simulink model "buck_boost_SMC"  (R2025a)
settings: Solver=ode3  StartTime=0.0  StopTime=1  FixedStep=1e-3  RelTol=1e-3  EnableMultiTasking=on
values from neighbouring files (symbols this model uses):
  beta = 2e3    (= 2000)    [projeakt_3.m]
  C = 470*10^-6    (= 0.00047)    [projeakt_3.m]
  den_NF = [1/800 1]    [projeakt_3.m]
  E = 12    [projeakt_3.m]
  k0 = 4*30    (= 120)    [projeakt_3.m]
  k1 = 1    [projeakt_3.m]
  ki = 4*30^2    (= 3600)    [projeakt_3.m]
  L = Ls(i)*15.91e-3    [projeakt_3.m]
  noise_var = 0    [projeakt_3.m]
  num_NF = [1]    [projeakt_3.m]
  R = 52    [projeakt_3.m]
  sel = 3    [projeakt_3.m]
  x2e = Vc    (= -22.5)    [projeakt_3.m]
settings Model: Creator=Stevica  LastModifiedBy=PC
settings SolverCC: AlgebraicLoopSolver=TrustRegion
settings DataIOCC: LimitDataPoints=on  SaveFormat=Array  ReturnWorkspaceOutputs=off
settings OptimizationCC: LifeSpan=inf
settings DebuggingCC: UnderspecifiedInitializationDetection=Classic  MergeDetectMultiDrivingBlocksExec=none  SolverPrmCheckMsg=warning  UnconnectedInputMsg=warning  UnconnectedOutputMsg=warning  UnconnectedLineMsg=warning  SFUnexpectedBacktrackingDiag=warning  SFNoUnconditionalDefaultTransitionDiag=warning  SFExecutionAtInitializationDiag=none  ArithmeticOperatorsInVariantConditions=warning
settings HardwareCC: ProdBitPerPointer=32.0  ProdBitPerSizeT=32.0  ProdBitPerPtrDiffT=32.0  ProdLargestAtomicFloat=None  ProdIntDivRoundTo=Undefined  ProdEndianess=Unspecified  ProdWordSize=32.0  ProdHWDeviceType=32-bit Generic
settings ModelReferenceCC: PropagateSignalLabelsOutOfModel=off
settings SFSimCC: SimUseLocalCustomCode=off  CustomCodeUndefinedFunction=UseInterfaceOnly
settings RTWCC: RTWUseLocalCustomCode=off  GPUComputeCapability=3.5
settings CodeAppCC: StateflowObjectComments=on
settings GRTTargetCC: TargetLangStandard=C89/C90 (ANSI)
settings ConfigComp: CovMetricSettings=dw  CovSaveCumulativeToWorkspaceVar=on  CovSaveSingleToWorkspaceVar=on  CovExternalEMLEnable=off

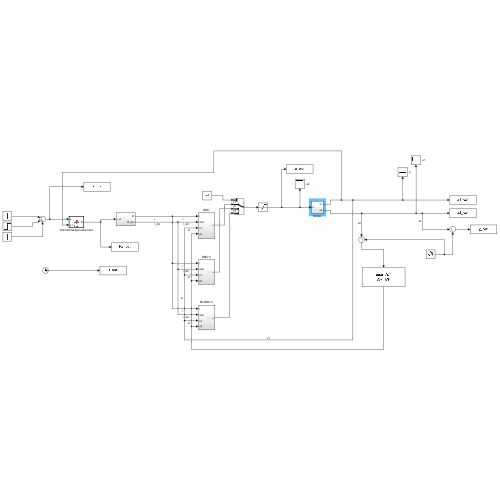
[thumbnail: Simulink's stored preview of the top-level diagram]
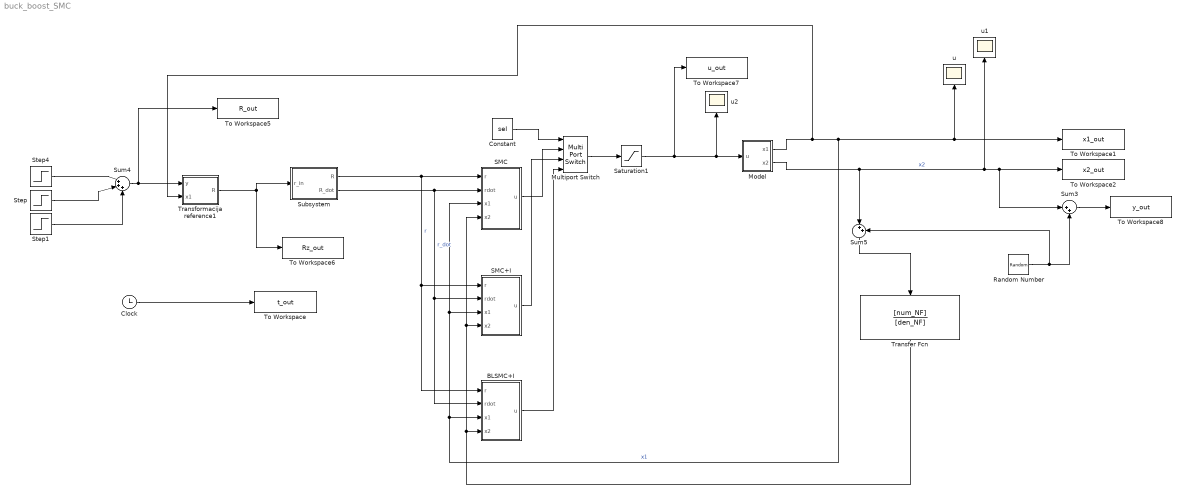
== system buck_boost_SMC ==
  BLSMC+I : Subsystem
      settings: PortSchema="{\"entries\":[{\"content\":{\"sides\":[{\"content\":{\"connectorIds\":[\"Out1\"]},\"type\":\"ConnectorPlacement.EquallySpacedRectSide\",\"uuid\":\"fc4d1246-7468-4525-a5ed-aeaa813f79b9\"},{\"content\":{\"connectorIds\":[\"In1\",\"In2\",\"In3\",\"In4\"],\"side\":\"RIGHT\"},\"type\":\"ConnectorPlacement.EquallySpacedRectSide\",\"uuid\":\"043d6a8f-e326-4119-9507-3ed5a55de0f4\"},{\"content\":{\"side\":\"TOP\"},\"type\":\"ConnectorPlacement.EquallySpacedRectSide\",\"uuid\":\"52d26304-56e6-4b52-8faf-a8e357024c95\"}]},\"type\":\"ConnectorPlacement.EquallySpacedConnector\",\"uuid\":\"d1c4fd68-439c-47cf-b9bf-33c74b646101\"}],\"packageUris\":[\"http://schema.mathworks.com/mf0/Connector/R2020b\"],\"version\":\"1.0\"}"
  Clock : Clock
  Constant : Constant  Value=sel
  Model : Subsystem
  Multiport Switch : MultiPortSwitch  SaturateOnIntegerOverflow=off  InputSameDT=off
  Random Number : RandomNumber  Variance=noise_var  SampleTime=0.001
  SMC : Subsystem
      settings: PortSchema="{\"entries\":[{\"content\":{\"sides\":[{\"content\":{\"connectorIds\":[\"Out1\"]},\"type\":\"ConnectorPlacement.EquallySpacedRectSide\",\"uuid\":\"fc4d1246-7468-4525-a5ed-aeaa813f79b9\"},{\"content\":{\"connectorIds\":[\"In1\",\"In2\",\"In3\",\"In4\"],\"side\":\"RIGHT\"},\"type\":\"ConnectorPlacement.EquallySpacedRectSide\",\"uuid\":\"043d6a8f-e326-4119-9507-3ed5a55de0f4\"},{\"content\":{\"side\":\"TOP\"},\"type\":\"ConnectorPlacement.EquallySpacedRectSide\",\"uuid\":\"52d26304-56e6-4b52-8faf-a8e357024c95\"}]},\"type\":\"ConnectorPlacement.EquallySpacedConnector\",\"uuid\":\"d1c4fd68-439c-47cf-b9bf-33c74b646101\"}],\"packageUris\":[\"http://schema.mathworks.com/mf0/Connector/R2020b\"],\"version\":\"1.0\"}"
  SMC+I : Subsystem
      settings: PortSchema="{\"entries\":[{\"content\":{\"sides\":[{\"content\":{\"connectorIds\":[\"Out1\"]},\"type\":\"ConnectorPlacement.EquallySpacedRectSide\",\"uuid\":\"fc4d1246-7468-4525-a5ed-aeaa813f79b9\"},{\"content\":{\"connectorIds\":[\"In1\",\"In2\",\"In3\",\"In4\"],\"side\":\"RIGHT\"},\"type\":\"ConnectorPlacement.EquallySpacedRectSide\",\"uuid\":\"043d6a8f-e326-4119-9507-3ed5a55de0f4\"},{\"content\":{\"side\":\"TOP\"},\"type\":\"ConnectorPlacement.EquallySpacedRectSide\",\"uuid\":\"52d26304-56e6-4b52-8faf-a8e357024c95\"}]},\"type\":\"ConnectorPlacement.EquallySpacedConnector\",\"uuid\":\"d1c4fd68-439c-47cf-b9bf-33c74b646101\"}],\"packageUris\":[\"http://schema.mathworks.com/mf0/Connector/R2020b\"],\"version\":\"1.0\"}"
  Saturation1 : Saturate  UpperLimit=0.9  LowerLimit=0.2
  Step : Step  Time=0.7  After=5  SampleTime=0
  Step1 : Step  Time=1.3  After=-5  SampleTime=0
  Step4 : Step  Time=0  After=x2e  SampleTime=0
  Subsystem : Subsystem
  Sum3 : Sum  Inputs=|++
  Sum4 : Sum  Inputs=|+++
  Sum5 : Sum  Inputs=|++
  To Workspace : ToWorkspace  VariableName=t_out  SampleTime=-1
  To Workspace1 : ToWorkspace  VariableName=x1_out  SampleTime=-1
  To Workspace2 : ToWorkspace  VariableName=x2_out  SampleTime=-1
  To Workspace5 : ToWorkspace  VariableName=R_out  SampleTime=-1
  To Workspace6 : ToWorkspace  VariableName=Rz_out  SampleTime=-1
  To Workspace7 : ToWorkspace  VariableName=u_out  SampleTime=-1
  To Workspace8 : ToWorkspace  VariableName=y_out  SampleTime=-1
  Transfer Fcn : TransferFcn  Numerator=[num_NF]  Denominator=[den_NF]
  Transformacija reference1 : MATLAB Function  TreatAsAtomicUnit=on
  u : Scope
      settings: ActiveDisplayYMinimum=-22.500000000014424  ActiveDisplayYMaximum=-22.49999999997209
  u1 : Scope
      settings: ActiveDisplayYMinimum=-22.174112994796246  ActiveDisplayYMaximum=-1.6560497868872126
  u2 : Scope
      settings: ActiveDisplayYMinimum=0.24319050212195464  ActiveDisplayYMaximum=1.29171952407274  DataLoggingVariableName=ScopeData3
  wires:
  Saturation1/1 -> Model/1(u), u2/1, To Workspace7/1
  Step/1 -> Sum4/2
  Step1/1 -> Sum4/3
  Model/1(x1) -> Transformacija reference1/2(x1), To Workspace1/1, u/1, BLSMC+I/3(x1), SMC/3(x1), SMC+I/3(x1)  "x1"
  Step4/1 -> Sum4/1
  SMC/1(u) -> Multiport Switch/2
  Multiport Switch/1 -> Saturation1/1
  Transformacija reference1/1(R) -> Subsystem/1(r_in), To Workspace6/1
  Subsystem/1(R) -> BLSMC+I/1(r), SMC+I/1(r), SMC/1(r)  "r"
  Subsystem/2(R_dot) -> BLSMC+I/2(rdot), SMC+I/2(rdot), SMC/2(rdot)  "r_dot"
  SMC+I/1(u) -> Multiport Switch/3
  BLSMC+I/1(u) -> Multiport Switch/4
  Constant/1 -> Multiport Switch/1
  Clock/1 -> To Workspace/1
  Sum4/1 -> Transformacija reference1/1(y), To Workspace5/1
  Model/2(x2) -> Sum3/1, To Workspace2/1, u1/1, Sum5/1  "x2"
  Random Number/1 -> Sum5/2, Sum3/2
  Sum3/1 -> To Workspace8/1
  Sum5/1 -> Transfer Fcn/1
  Transfer Fcn/1 -> SMC/4(x2), SMC+I/4(x2), BLSMC+I/4(x2)

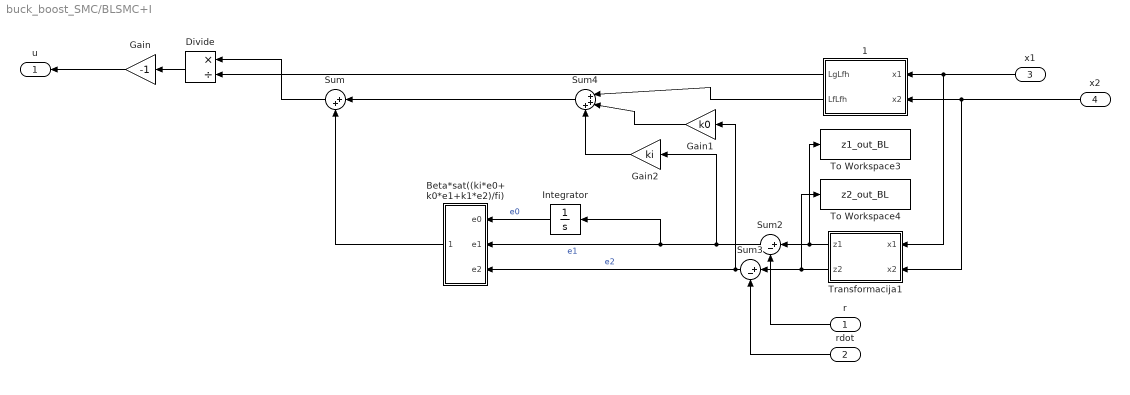
== system buck_boost_SMC/BLSMC+I ==
  r : Inport
  rdot : Inport  Port=2
  x1 : Inport  Port=3
  x2 : Inport  Port=4
  " 1" : MATLAB Function  TreatAsAtomicUnit=on
  Beta*sat((ki*e0+ k0*e1+k1*e2)/fi) : Subsystem
  Divide : Product  Inputs=*/
  Gain : Gain  Gain=-1
  Gain1 : Gain  Gain=k0
  Gain2 : Gain  Gain=ki
  Integrator : Integrator
  Sum : Sum  Inputs=|++
  Sum2 : Sum  Inputs=|+-
  Sum3 : Sum  Inputs=|+-
  Sum4 : Sum  Inputs=|+++
  To Workspace3 : ToWorkspace  VariableName=z1_out_BL  SampleTime=-1
  To Workspace4 : ToWorkspace  VariableName=z2_out_BL  SampleTime=-1
  Transformacija1 : MATLAB Function  TreatAsAtomicUnit=on
  u : Outport
  wires:
  x1/1 -> Transformacija1/1(x1), " 1"/1(x1)
  x2/1 -> Transformacija1/2(x2), " 1"/2(x2)
  Sum3/1 -> Gain1/1, Beta*sat((ki*e0+ k0*e1+k1*e2)/fi)/3(e2)  "e2"
  rdot/1 -> Sum3/2
  " 1"/2(LfLfh) -> Sum4/1
  Gain1/1 -> Sum4/2
  Sum4/1 -> Sum/1
  Sum2/1 -> Gain2/1, Beta*sat((ki*e0+ k0*e1+k1*e2)/fi)/2(e1), Integrator/1  "e1"
  Beta*sat((ki*e0+ k0*e1+k1*e2)/fi)/1(Out1) -> Sum/2
  Sum/1 -> Divide/1
  " 1"/1(LgLfh) -> Divide/2
  Divide/1 -> Gain/1
  Gain/1 -> u/1
  Integrator/1 -> Beta*sat((ki*e0+ k0*e1+k1*e2)/fi)/1(e0)  "e0"
  Gain2/1 -> Sum4/3
  Transformacija1/2(z2) -> To Workspace4/1, Sum3/1
  r/1 -> Sum2/2
  Transformacija1/1(z1) -> Sum2/1, To Workspace3/1

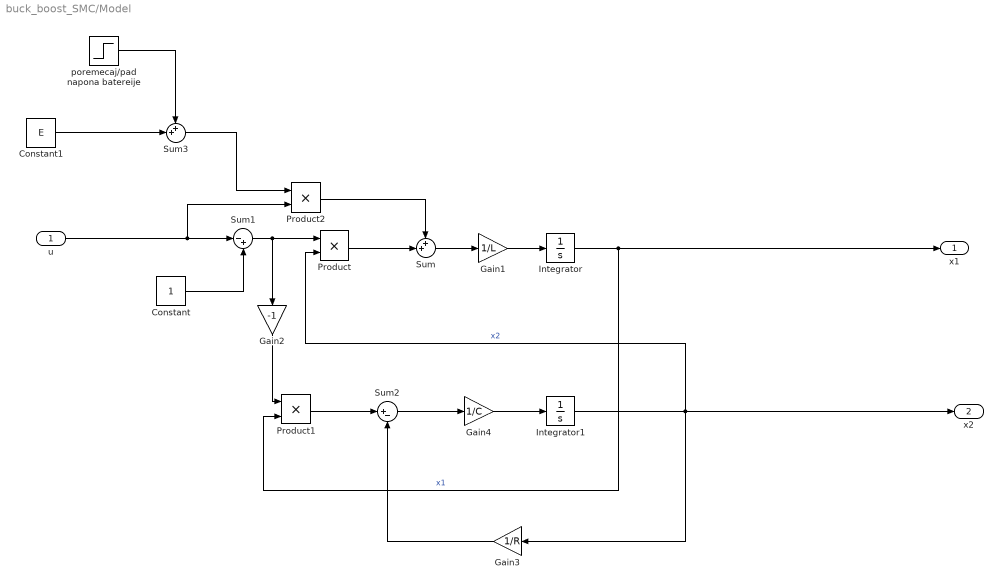
== system buck_boost_SMC/Model ==
  u : Inport
  Constant : Constant
  Constant1 : Constant  Value=E
  Gain1 : Gain  Gain=1/L
  Gain2 : Gain  Gain=-1
  Gain3 : Gain  Gain=1/R
  Gain4 : Gain  Gain=1/C
  Integrator : Integrator  LimitOutput=on  LowerSaturationLimit=0
  Integrator1 : Integrator  LimitOutput=on  UpperSaturationLimit=0
  Product : Product
  Product1 : Product
  Product2 : Product
  Sum : Sum  Inputs=++|
  Sum1 : Sum  Inputs=|-+
  Sum2 : Sum  Inputs=|+-
  Sum3 : Sum  Inputs=++|
  poremecaj/pad napona batereije : Step  Time=1.9  After=-1  SampleTime=0
  x1 : Outport
  x2 : Outport  Port=2
  wires:
  Product1/1 -> Sum2/1
  Integrator1/1 -> x2/1, Gain3/1, Product/2  "x2"
  Gain3/1 -> Sum2/2
  Constant/1 -> Sum1/2
  Sum2/1 -> Gain4/1
  Product/1 -> Sum/2
  Gain1/1 -> Integrator/1
  Sum1/1 -> Product/1, Gain2/1
  Integrator/1 -> x1/1, Product1/2  "x1"
  Product2/1 -> Sum/1
  u/1 -> Product2/2, Sum1/1
  Gain4/1 -> Integrator1/1
  Sum/1 -> Gain1/1
  Gain2/1 -> Product1/1
  Constant1/1 -> Sum3/2
  poremecaj/pad napona batereije/1 -> Sum3/1
  Sum3/1 -> Product2/1

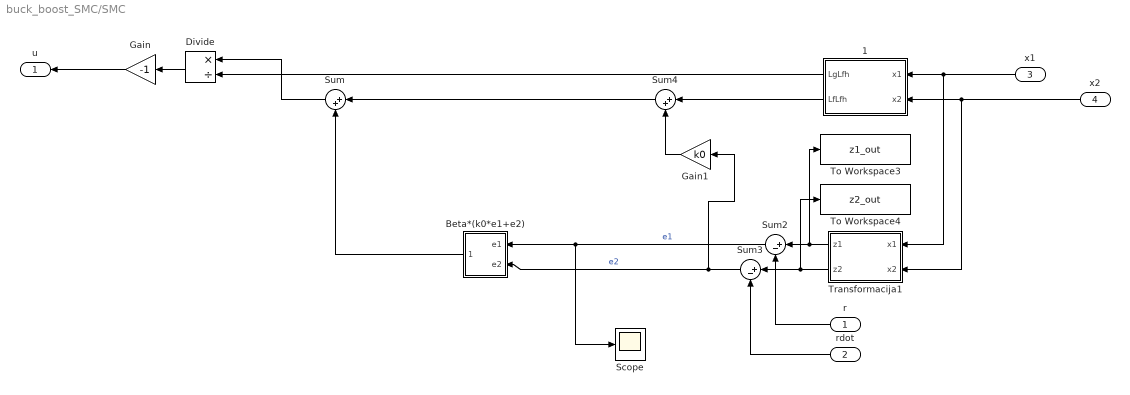
== system buck_boost_SMC/SMC ==
  r : Inport
  rdot : Inport  Port=2
  x1 : Inport  Port=3
  x2 : Inport  Port=4
  " 1" : MATLAB Function  TreatAsAtomicUnit=on
  Beta*(k0*e1+e2) : Subsystem
  Divide : Product  Inputs=*/
  Gain : Gain  Gain=-1
  Gain1 : Gain  Gain=k0
  Scope : Scope
      settings: ActiveDisplayYMinimum=-0.069567507965081155  ActiveDisplayYMaximum=0.050581461220904358  DataLoggingVariableName=ScopeData5
  Sum : Sum  Inputs=|++
  Sum2 : Sum  Inputs=|+-
  Sum3 : Sum  Inputs=|+-
  Sum4 : Sum  Inputs=|++
  To Workspace3 : ToWorkspace  VariableName=z1_out  SampleTime=-1
  To Workspace4 : ToWorkspace  VariableName=z2_out  SampleTime=-1
  Transformacija1 : MATLAB Function  TreatAsAtomicUnit=on
  u : Outport
  wires:
  Transformacija1/1(z1) -> To Workspace3/1, Sum2/1
  x1/1 -> " 1"/1(x1), Transformacija1/1(x1)
  x2/1 -> " 1"/2(x2), Transformacija1/2(x2)
  Transformacija1/2(z2) -> To Workspace4/1, Sum3/1
  Sum3/1 -> Beta*(k0*e1+e2)/2(e2), Gain1/1  "e2"
  r/1 -> Sum2/2
  rdot/1 -> Sum3/2
  " 1"/2(LfLfh) -> Sum4/1
  Gain1/1 -> Sum4/2
  Sum4/1 -> Sum/1
  Sum2/1 -> Scope/1, Beta*(k0*e1+e2)/1(e1)  "e1"
  Beta*(k0*e1+e2)/1(Out1) -> Sum/2
  Sum/1 -> Divide/1
  " 1"/1(LgLfh) -> Divide/2
  Divide/1 -> Gain/1
  Gain/1 -> u/1

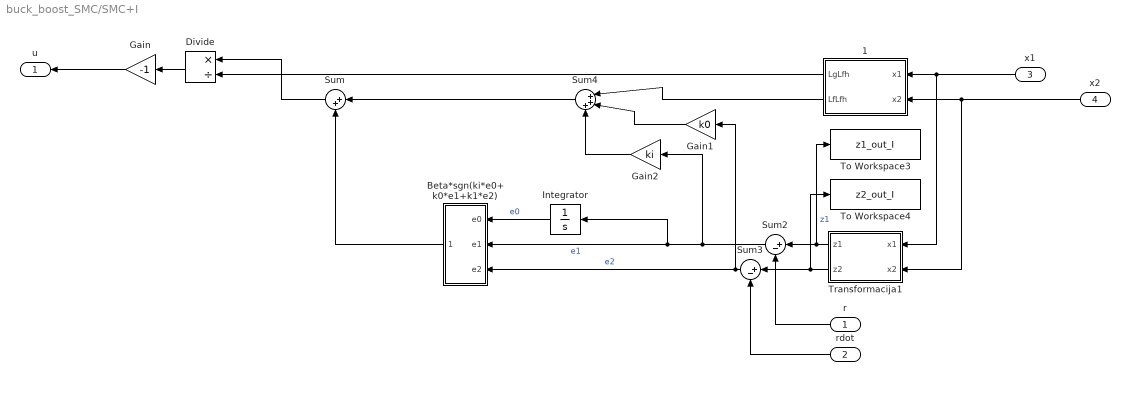
== system buck_boost_SMC/SMC+I ==
  r : Inport
  rdot : Inport  Port=2
  x1 : Inport  Port=3
  x2 : Inport  Port=4
  " 1" : MATLAB Function  TreatAsAtomicUnit=on
  Beta*sgn(ki*e0+ k0*e1+k1*e2) : Subsystem
  Divide : Product  Inputs=*/
  Gain : Gain  Gain=-1
  Gain1 : Gain  Gain=k0
  Gain2 : Gain  Gain=ki
  Integrator : Integrator
  Sum : Sum  Inputs=|++
  Sum2 : Sum  Inputs=|+-
  Sum3 : Sum  Inputs=|+-
  Sum4 : Sum  Inputs=|+++
  To Workspace3 : ToWorkspace  VariableName=z1_out_I  SampleTime=-1
  To Workspace4 : ToWorkspace  VariableName=z2_out_I  SampleTime=-1
  Transformacija1 : MATLAB Function  TreatAsAtomicUnit=on
  u : Outport
  wires:
  x1/1 -> " 1"/1(x1), Transformacija1/1(x1)
  x2/1 -> " 1"/2(x2), Transformacija1/2(x2)
  Sum3/1 -> Gain1/1, Beta*sgn(ki*e0+ k0*e1+k1*e2)/3(e2)  "e2"
  r/1 -> Sum2/2
  rdot/1 -> Sum3/2
  " 1"/2(LfLfh) -> Sum4/1
  Gain1/1 -> Sum4/2
  Sum4/1 -> Sum/1
  Sum2/1 -> Gain2/1, Beta*sgn(ki*e0+ k0*e1+k1*e2)/2(e1), Integrator/1  "e1"
  Beta*sgn(ki*e0+ k0*e1+k1*e2)/1(Out1) -> Sum/2
  Sum/1 -> Divide/1
  " 1"/1(LgLfh) -> Divide/2
  Divide/1 -> Gain/1
  Gain/1 -> u/1
  Integrator/1 -> Beta*sgn(ki*e0+ k0*e1+k1*e2)/1(e0)  "e0"
  Gain2/1 -> Sum4/3
  Transformacija1/2(z2) -> To Workspace4/1, Sum3/1
  Transformacija1/1(z1) -> To Workspace3/1, Sum2/1  "z1"

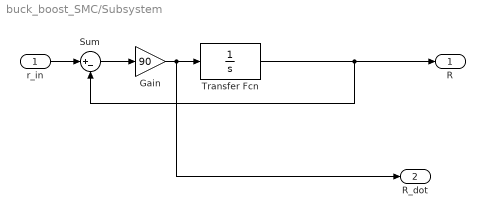
== system buck_boost_SMC/Subsystem ==
  r_in : Inport
  Gain : Gain  Gain=90
  Sum : Sum  Inputs=|+-
  Transfer Fcn : TransferFcn  Denominator=[1 0]
  R : Outport
  R_dot : Outport  Port=2
  wires:
  r_in/1 -> Sum/1
  Sum/1 -> Gain/1
  Transfer Fcn/1 -> Sum/2, R/1
  Gain/1 -> R_dot/1, Transfer Fcn/1

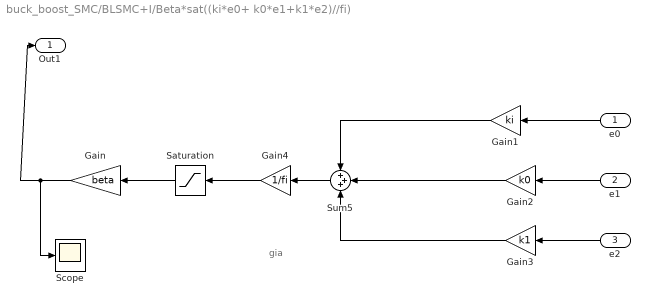
== system buck_boost_SMC/BLSMC+I/Beta*sat((ki*e0+ k0*e1+k1*e2)//fi) ==
  note: gia
  e0 : Inport
  e1 : Inport  Port=2
  e2 : Inport  Port=3
  Gain : Gain  Gain=beta
  Gain1 : Gain  Gain=ki
  Gain2 : Gain  Gain=k0
  Gain3 : Gain  Gain=k1
  Gain4 : Gain  Gain=1/fi
  Saturation : Saturate  UpperLimit=1  LowerLimit=-1
  Scope : Scope
      settings: ActiveDisplayYMinimum=-6728.468140991592  ActiveDisplayYMaximum=8629.1506385974171  DataLoggingVariableName=ScopeData4
  Sum5 : Sum  Inputs=+++
  Out1 : Outport
  wires:
  Gain2/1 -> Sum5/2
  Sum5/1 -> Gain4/1
  Saturation/1 -> Gain/1
  e1/1 -> Gain2/1
  Gain/1 -> Scope/1, Out1/1
  e2/1 -> Gain3/1
  e0/1 -> Gain1/1
  Gain1/1 -> Sum5/1
  Gain3/1 -> Sum5/3
  Gain4/1 -> Saturation/1

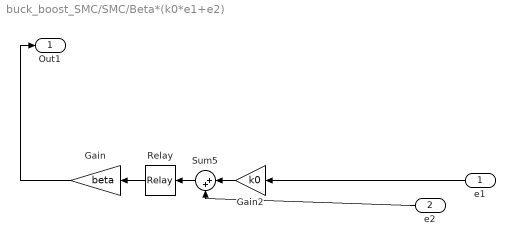
== system buck_boost_SMC/SMC/Beta*(k0*e1+e2) ==
  e1 : Inport
  e2 : Inport  Port=2
  Gain : Gain  Gain=beta
  Gain2 : Gain  Gain=k0
  Relay : Relay  OnSwitchValue=0  OffSwitchValue=0  OffOutputValue=-1
  Sum5 : Sum  Inputs=|++
  Out1 : Outport
  wires:
  Gain2/1 -> Sum5/1
  Sum5/1 -> Relay/1
  Relay/1 -> Gain/1
  e1/1 -> Gain2/1
  Gain/1 -> Out1/1
  e2/1 -> Sum5/2

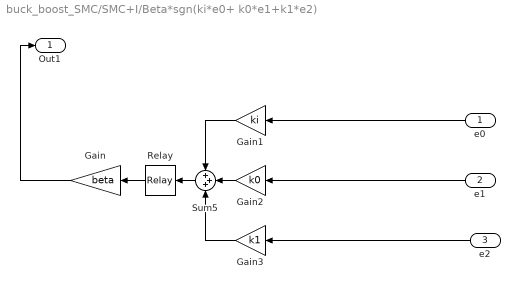
== system buck_boost_SMC/SMC+I/Beta*sgn(ki*e0+ k0*e1+k1*e2) ==
  e0 : Inport
  e1 : Inport  Port=2
  e2 : Inport  Port=3
  Gain : Gain  Gain=beta
  Gain1 : Gain  Gain=ki
  Gain2 : Gain  Gain=k0
  Gain3 : Gain  Gain=k1
  Relay : Relay  OnSwitchValue=0  OffSwitchValue=0  OffOutputValue=-1
  Sum5 : Sum  Inputs=+++
  Out1 : Outport
  wires:
  Gain2/1 -> Sum5/2
  Sum5/1 -> Relay/1
  Relay/1 -> Gain/1
  e1/1 -> Gain2/1
  Gain/1 -> Out1/1
  e2/1 -> Gain3/1
  e0/1 -> Gain1/1
  Gain1/1 -> Sum5/1
  Gain3/1 -> Sum5/3

== matlab function buck_boost_SMC/SMC/ 1 ==
  data: x1 input; LgLfh output; x2 input; LfLfh output
function [LgLfh, LfLfh] = fcn(x1, x2)

L=15.91*10^-3;
C=470*10^-6;
R=52;
E=12;

LgLfh = -4/(R*C)*x1*x2 + 2*E/(R*C)*x1 + 2*E^2/L - 2*E/L*x2;
LfLfh = 4/(R^2*C)*x2^2 - 2*E/(R^2*C)*x2 + 2*E/L*x2 - 2*E/(R*C)*x1 +4/(R*C)*x1*x2;

== matlab function buck_boost_SMC/SMC+I/Transformacija1 ==
  data: x1 input; z1 output; x2 input; z2 output
function [z1, z2] = fcn(x1, x2)

L=15.91*10^-3;
C=470*10^-6;
R=52;
E=12;

Vc=-22.5;
x2e=Vc;
x1e=1.2441;


z1 = C*x2^2 - 2*E*C*x2 + L*x1^2 - (C*x2e^2 - 2*E*C*x2e + L*x1e^2);
z2 = -2/R*x2^2 + 2*E*x1 + 2*E/R*x2;

== matlab function buck_boost_SMC/BLSMC+I/ 1 ==
  data: x1 input; LgLfh output; x2 input; LfLfh output
function [LgLfh, LfLfh] = fcn(x1, x2)

L=15.91*10^-3;
C=470*10^-6;
R=52;
E=12;

LgLfh = -4/(R*C)*x1*x2 + 2*E/(R*C)*x1 + 2*E^2/L - 2*E/L*x2;
LfLfh = 4/(R^2*C)*x2^2 - 2*E/(R^2*C)*x2 + 2*E/L*x2 - 2*E/(R*C)*x1 +4/(R*C)*x1*x2;

== matlab function buck_boost_SMC/SMC+I/ 1 ==
  data: x1 input; LgLfh output; x2 input; LfLfh output
function [LgLfh, LfLfh] = fcn(x1, x2)

L=15.91*10^-3;
C=470*10^-6;
R=52;
E=12;

LgLfh = -4/(R*C)*x1*x2 + 2*E/(R*C)*x1 + 2*E^2/L - 2*E/L*x2;
LfLfh = 4/(R^2*C)*x2^2 - 2*E/(R^2*C)*x2 + 2*E/L*x2 - 2*E/(R*C)*x1 +4/(R*C)*x1*x2;

== matlab function buck_boost_SMC/BLSMC+I/Transformacija1 ==
  data: x1 input; z1 output; x2 input; z2 output
function [z1, z2] = fcn(x1, x2)

L=15.91*10^-3;
C=470*10^-6;
R=52;
E=12;

Vc=-22.5;
x2e=Vc;
x1e=1.2441;


z1 = C*x2^2 - 2*E*C*x2 + L*x1^2 - (C*x2e^2 - 2*E*C*x2e + L*x1e^2);
z2 = -2/R*x2^2 + 2*E*x1 + 2*E/R*x2;

== matlab function buck_boost_SMC/Transformacija reference1 ==
  data: y input; R output; x1 input
function  R= fcn(y,x1)

% y=x1e stara referenca, tj. nominalna vrednost

L=15.91*10^-3;
C=470*10^-6;
R=52;
E=12;

Vc=-22.5;
x2e=Vc;
x1e=1.2441;

gama = C*x2e^2 - 2*E*C*x2e + L*x1e^2;

R = C*y^2 - 2*E*C*y + L*(x1)^2 - gama;

== matlab function buck_boost_SMC/SMC/Transformacija1 ==
  data: x1 input; z1 output; x2 input; z2 output
function [z1, z2] = fcn(x1, x2)

L=15.91*10^-3;
C=470*10^-6;
R=52;
E=12;

Vc=-22.5;
x2e=Vc;
x1e=1.2441;


z1 = C*x2^2 - 2*E*C*x2 + L*x1^2 - (C*x2e^2 - 2*E*C*x2e + L*x1e^2);
z2 = -2/R*x2^2 + 2*E*x1 + 2*E/R*x2;
